simulink model "c00014M_harness"  (R2018a)
settings: Solver=FixedStepAuto  StartTime=0.0  StopTime=300  FixedStep=0.1  RelTol=1e-3
undefined symbols (not defined in the file): A1, hmax, PriorityTank, R1, R2, sigbuilder_block
(part 9 of 24)

== system c00014M_harness/M236/Tank3 ==
  CT3 : Inport
  T3 : Inport  Port=2
  EB3 : Inport  Port=3
  LL1 : Inport  Port=4
  Control : Subsystem
  Logical Operator : Logic  AllPortsSameDT=off  OutDataTypeStr=boolean
  MasterTankControl : Subsystem
  Memory : Memory
  Memory1 : Memory
  TankModel : Subsystem
  LL3 : Outport
  wires:
  TankModel/1(LiquidLevel) -> Memory/1, LL3/1
  Control/1(LiquidIn) -> Logical Operator/1
  Control/2(LiquidOut) -> TankModel/2(LiquidOut)
  Memory/1 -> MasterTankControl/2(LiquidTank3), Control/4(LiquidLevel)
  CT3/1 -> Control/2(StartMaintenance), Control/1(ControlType)
  Memory1/1 -> MasterTankControl/1(LiquidTank1)
  EB3/1 -> Control/3(EmergencyButton)
  MasterTankControl/1(AllowTheTankFilling) -> Logical Operator/2
  Logical Operator/1 -> TankModel/1(LiquidIn)
  LL1/1 -> Memory1/1

== system c00014M_harness/M237/Tank1 ==
  CT1 : Inport
  F1 : Inport  Port=2
  E1 : Inport  Port=3
  T1 : Inport  Port=4
  EB1 : Inport  Port=5
  LL3 : Inport  Port=6
  Control : Subsystem
  Logical Operator : Logic  AllPortsSameDT=off  OutDataTypeStr=boolean
  MasterTankControl : Subsystem
  Memory : Memory
  Memory2 : Memory
  TankModel : Subsystem
  LL1 : Outport
  wires:
  TankModel/1(LiquidLevel) -> Memory/1, LL1/1
  Control/1(LiquidIn) -> Logical Operator/1
  Control/2(LiquidOut) -> TankModel/2(LiquidOut)
  Memory/1 -> Control/5(LiquidLevel), MasterTankControl/1(LiquidTank1)
  CT1/1 -> Control/1(ControlType)
  F1/1 -> Control/2(Fill)
  E1/1 -> Control/3(Empty)
  LL3/1 -> Memory2/1
  Memory2/1 -> MasterTankControl/2(LiquidTank3)
  EB1/1 -> Control/4(EmergencyButton)
  MasterTankControl/1(AllowTheTankFilling) -> Logical Operator/2
  Logical Operator/1 -> TankModel/1(LiquidIn)

== system c00014M_harness/M237/Tank3 ==
  CT3 : Inport
  T3 : Inport  Port=2
  EB3 : Inport  Port=3
  LL1 : Inport  Port=4
  Control : Subsystem
  Logical Operator : Logic  AllPortsSameDT=off  OutDataTypeStr=boolean
  MasterTankControl : Subsystem
  Memory : Memory
  Memory1 : Memory
  TankModel : Subsystem
  LL3 : Outport
  wires:
  TankModel/1(LiquidLevel) -> Memory/1, LL3/1
  Control/1(LiquidIn) -> Logical Operator/1
  Control/2(LiquidOut) -> TankModel/2(LiquidOut)
  Memory/1 -> MasterTankControl/2(LiquidTank3), Control/4(LiquidLevel)
  CT3/1 -> Control/2(StartMaintenance), Control/1(ControlType)
  Memory1/1 -> MasterTankControl/1(LiquidTank1)
  EB3/1 -> Control/3(EmergencyButton)
  MasterTankControl/1(AllowTheTankFilling) -> Logical Operator/2
  Logical Operator/1 -> TankModel/1(LiquidIn)
  LL1/1 -> Memory1/1

== system c00014M_harness/M238/Tank1 ==
  CT1 : Inport
  F1 : Inport  Port=2
  E1 : Inport  Port=3
  T1 : Inport  Port=4
  EB1 : Inport  Port=5
  LL3 : Inport  Port=6
  Control : Subsystem
  Logical Operator : Logic  AllPortsSameDT=off  OutDataTypeStr=boolean
  MasterTankControl : Subsystem
  Memory : Memory
  Memory2 : Memory
  TankModel : Subsystem
  LL1 : Outport
  wires:
  TankModel/1(LiquidLevel) -> Memory/1, LL1/1
  Control/1(LiquidIn) -> Logical Operator/1
  Control/2(LiquidOut) -> TankModel/2(LiquidOut)
  Memory/1 -> Control/5(LiquidLevel), MasterTankControl/1(LiquidTank1)
  CT1/1 -> Control/1(ControlType)
  F1/1 -> Control/2(Fill)
  E1/1 -> Control/3(Empty)
  LL3/1 -> Memory2/1
  Memory2/1 -> MasterTankControl/2(LiquidTank3)
  EB1/1 -> Control/4(EmergencyButton)
  MasterTankControl/1(AllowTheTankFilling) -> Logical Operator/2
  Logical Operator/1 -> TankModel/1(LiquidIn)

== system c00014M_harness/M238/Tank3 ==
  CT3 : Inport
  T3 : Inport  Port=2
  EB3 : Inport  Port=3
  LL1 : Inport  Port=4
  Control : Subsystem
  Logical Operator : Logic  AllPortsSameDT=off  OutDataTypeStr=boolean
  MasterTankControl : Subsystem
  Memory : Memory
  Memory1 : Memory
  TankModel : Subsystem
  LL3 : Outport
  wires:
  TankModel/1(LiquidLevel) -> Memory/1, LL3/1
  Control/1(LiquidIn) -> Logical Operator/1
  Control/2(LiquidOut) -> TankModel/2(LiquidOut)
  Memory/1 -> MasterTankControl/2(LiquidTank3), Control/4(LiquidLevel)
  CT3/1 -> Control/2(StartMaintenance), Control/1(ControlType)
  Memory1/1 -> MasterTankControl/1(LiquidTank1)
  EB3/1 -> Control/3(EmergencyButton)
  MasterTankControl/1(AllowTheTankFilling) -> Logical Operator/2
  Logical Operator/1 -> TankModel/1(LiquidIn)
  LL1/1 -> Memory1/1

== system c00014M_harness/M239/Tank1 ==
  CT1 : Inport
  F1 : Inport  Port=2
  E1 : Inport  Port=3
  T1 : Inport  Port=4
  EB1 : Inport  Port=5
  LL3 : Inport  Port=6
  Control : Subsystem
  Logical Operator : Logic  AllPortsSameDT=off  OutDataTypeStr=boolean
  MasterTankControl : Subsystem
  Memory : Memory
  Memory2 : Memory
  TankModel : Subsystem
  LL1 : Outport
  wires:
  TankModel/1(LiquidLevel) -> Memory/1, LL1/1
  Control/1(LiquidIn) -> Logical Operator/1
  Control/2(LiquidOut) -> TankModel/2(LiquidOut)
  Memory/1 -> Control/5(LiquidLevel), MasterTankControl/1(LiquidTank1)
  CT1/1 -> Control/1(ControlType)
  F1/1 -> Control/2(Fill)
  E1/1 -> Control/3(Empty)
  LL3/1 -> Memory2/1
  Memory2/1 -> MasterTankControl/2(LiquidTank3)
  EB1/1 -> Control/4(EmergencyButton)
  MasterTankControl/1(AllowTheTankFilling) -> Logical Operator/2
  Logical Operator/1 -> TankModel/1(LiquidIn)

== system c00014M_harness/M239/Tank3 ==
  CT3 : Inport
  T3 : Inport  Port=2
  EB3 : Inport  Port=3
  LL1 : Inport  Port=4
  Control : Subsystem
  Logical Operator : Logic  AllPortsSameDT=off  OutDataTypeStr=boolean
  MasterTankControl : Subsystem
  Memory : Memory
  Memory1 : Memory
  TankModel : Subsystem
  LL3 : Outport
  wires:
  TankModel/1(LiquidLevel) -> Memory/1, LL3/1
  Control/1(LiquidIn) -> Logical Operator/1
  Control/2(LiquidOut) -> TankModel/2(LiquidOut)
  Memory/1 -> MasterTankControl/2(LiquidTank3), Control/4(LiquidLevel)
  CT3/1 -> Control/2(StartMaintenance), Control/1(ControlType)
  Memory1/1 -> MasterTankControl/1(LiquidTank1)
  EB3/1 -> Control/3(EmergencyButton)
  MasterTankControl/1(AllowTheTankFilling) -> Logical Operator/2
  Logical Operator/1 -> TankModel/1(LiquidIn)
  LL1/1 -> Memory1/1

== system c00014M_harness/M240/Tank1 ==
  CT1 : Inport
  F1 : Inport  Port=2
  E1 : Inport  Port=3
  T1 : Inport  Port=4
  EB1 : Inport  Port=5
  LL3 : Inport  Port=6
  Control : Subsystem
  Logical Operator : Logic  AllPortsSameDT=off  OutDataTypeStr=boolean
  MasterTankControl : Subsystem
  Memory : Memory
  Memory2 : Memory
  TankModel : Subsystem
  LL1 : Outport
  wires:
  TankModel/1(LiquidLevel) -> Memory/1, LL1/1
  Control/1(LiquidIn) -> Logical Operator/1
  Control/2(LiquidOut) -> TankModel/2(LiquidOut)
  Memory/1 -> Control/5(LiquidLevel), MasterTankControl/1(LiquidTank1)
  CT1/1 -> Control/1(ControlType)
  F1/1 -> Control/2(Fill)
  E1/1 -> Control/3(Empty)
  LL3/1 -> Memory2/1
  Memory2/1 -> MasterTankControl/2(LiquidTank3)
  EB1/1 -> Control/4(EmergencyButton)
  MasterTankControl/1(AllowTheTankFilling) -> Logical Operator/2
  Logical Operator/1 -> TankModel/1(LiquidIn)

== system c00014M_harness/M240/Tank3 ==
  CT3 : Inport
  T3 : Inport  Port=2
  EB3 : Inport  Port=3
  LL1 : Inport  Port=4
  Control : Subsystem
  Logical Operator : Logic  AllPortsSameDT=off  OutDataTypeStr=boolean
  MasterTankControl : Subsystem
  Memory : Memory
  Memory1 : Memory
  TankModel : Subsystem
  LL3 : Outport
  wires:
  TankModel/1(LiquidLevel) -> Memory/1, LL3/1
  Control/1(LiquidIn) -> Logical Operator/1
  Control/2(LiquidOut) -> TankModel/2(LiquidOut)
  Memory/1 -> MasterTankControl/2(LiquidTank3), Control/4(LiquidLevel)
  CT3/1 -> Control/2(StartMaintenance), Control/1(ControlType)
  Memory1/1 -> MasterTankControl/1(LiquidTank1)
  EB3/1 -> Control/3(EmergencyButton)
  MasterTankControl/1(AllowTheTankFilling) -> Logical Operator/2
  Logical Operator/1 -> TankModel/1(LiquidIn)
  LL1/1 -> Memory1/1

== system c00014M_harness/M241/Tank1 ==
  CT1 : Inport
  F1 : Inport  Port=2
  E1 : Inport  Port=3
  T1 : Inport  Port=4
  EB1 : Inport  Port=5
  LL3 : Inport  Port=6
  Control : Subsystem
  Logical Operator : Logic  AllPortsSameDT=off  OutDataTypeStr=boolean
  MasterTankControl : Subsystem
  Memory : Memory
  Memory2 : Memory
  TankModel : Subsystem
  LL1 : Outport
  wires:
  TankModel/1(LiquidLevel) -> Memory/1, LL1/1
  Control/1(LiquidIn) -> Logical Operator/1
  Control/2(LiquidOut) -> TankModel/2(LiquidOut)
  Memory/1 -> Control/5(LiquidLevel), MasterTankControl/1(LiquidTank1)
  CT1/1 -> Control/1(ControlType)
  F1/1 -> Control/2(Fill)
  E1/1 -> Control/3(Empty)
  LL3/1 -> Memory2/1
  Memory2/1 -> MasterTankControl/2(LiquidTank3)
  EB1/1 -> Control/4(EmergencyButton)
  MasterTankControl/1(AllowTheTankFilling) -> Logical Operator/2
  Logical Operator/1 -> TankModel/1(LiquidIn)

== system c00014M_harness/M241/Tank3 ==
  CT3 : Inport
  T3 : Inport  Port=2
  EB3 : Inport  Port=3
  LL1 : Inport  Port=4
  Control : Subsystem
  Logical Operator : Logic  AllPortsSameDT=off  OutDataTypeStr=boolean
  MasterTankControl : Subsystem
  Memory : Memory
  Memory1 : Memory
  TankModel : Subsystem
  LL3 : Outport
  wires:
  TankModel/1(LiquidLevel) -> Memory/1, LL3/1
  Control/1(LiquidIn) -> Logical Operator/1
  Control/2(LiquidOut) -> TankModel/2(LiquidOut)
  Memory/1 -> MasterTankControl/2(LiquidTank3), Control/4(LiquidLevel)
  CT3/1 -> Control/2(StartMaintenance), Control/1(ControlType)
  Memory1/1 -> MasterTankControl/1(LiquidTank1)
  EB3/1 -> Control/3(EmergencyButton)
  MasterTankControl/1(AllowTheTankFilling) -> Logical Operator/2
  Logical Operator/1 -> TankModel/1(LiquidIn)
  LL1/1 -> Memory1/1

== system c00014M_harness/M242/Tank1 ==
  CT1 : Inport
  F1 : Inport  Port=2
  E1 : Inport  Port=3
  T1 : Inport  Port=4
  EB1 : Inport  Port=5
  LL3 : Inport  Port=6
  Control : Subsystem
  Logical Operator : Logic  AllPortsSameDT=off  OutDataTypeStr=boolean
  MasterTankControl : Subsystem
  Memory : Memory
  Memory2 : Memory
  TankModel : Subsystem
  LL1 : Outport
  wires:
  TankModel/1(LiquidLevel) -> Memory/1, LL1/1
  Control/1(LiquidIn) -> Logical Operator/1
  Control/2(LiquidOut) -> TankModel/2(LiquidOut)
  Memory/1 -> Control/5(LiquidLevel), MasterTankControl/1(LiquidTank1)
  CT1/1 -> Control/1(ControlType)
  F1/1 -> Control/2(Fill)
  E1/1 -> Control/3(Empty)
  LL3/1 -> Memory2/1
  Memory2/1 -> MasterTankControl/2(LiquidTank3)
  EB1/1 -> Control/4(EmergencyButton)
  MasterTankControl/1(AllowTheTankFilling) -> Logical Operator/2
  Logical Operator/1 -> TankModel/1(LiquidIn)

== system c00014M_harness/M242/Tank3 ==
  CT3 : Inport
  T3 : Inport  Port=2
  EB3 : Inport  Port=3
  LL1 : Inport  Port=4
  Control : Subsystem
  Logical Operator : Logic  AllPortsSameDT=off  OutDataTypeStr=boolean
  MasterTankControl : Subsystem
  Memory : Memory
  Memory1 : Memory
  TankModel : Subsystem
  LL3 : Outport
  wires:
  TankModel/1(LiquidLevel) -> Memory/1, LL3/1
  Control/1(LiquidIn) -> Logical Operator/1
  Control/2(LiquidOut) -> TankModel/2(LiquidOut)
  Memory/1 -> MasterTankControl/2(LiquidTank3), Control/4(LiquidLevel)
  CT3/1 -> Control/2(StartMaintenance), Control/1(ControlType)
  Memory1/1 -> MasterTankControl/1(LiquidTank1)
  EB3/1 -> Control/3(EmergencyButton)
  MasterTankControl/1(AllowTheTankFilling) -> Logical Operator/2
  Logical Operator/1 -> TankModel/1(LiquidIn)
  LL1/1 -> Memory1/1

== system c00014M_harness/M243/Tank1 ==
  CT1 : Inport
  F1 : Inport  Port=2
  E1 : Inport  Port=3
  T1 : Inport  Port=4
  EB1 : Inport  Port=5
  LL3 : Inport  Port=6
  Control : Subsystem
  Logical Operator : Logic  AllPortsSameDT=off  OutDataTypeStr=boolean
  MasterTankControl : Subsystem
  Memory : Memory
  Memory2 : Memory
  TankModel : Subsystem
  LL1 : Outport
  wires:
  TankModel/1(LiquidLevel) -> Memory/1, LL1/1
  Control/1(LiquidIn) -> Logical Operator/1
  Control/2(LiquidOut) -> TankModel/2(LiquidOut)
  Memory/1 -> Control/5(LiquidLevel), MasterTankControl/1(LiquidTank1)
  CT1/1 -> Control/1(ControlType)
  F1/1 -> Control/2(Fill)
  E1/1 -> Control/3(Empty)
  LL3/1 -> Memory2/1
  Memory2/1 -> MasterTankControl/2(LiquidTank3)
  EB1/1 -> Control/4(EmergencyButton)
  MasterTankControl/1(AllowTheTankFilling) -> Logical Operator/2
  Logical Operator/1 -> TankModel/1(LiquidIn)

== system c00014M_harness/M243/Tank3 ==
  CT3 : Inport
  T3 : Inport  Port=2
  EB3 : Inport  Port=3
  LL1 : Inport  Port=4
  Control : Subsystem
  Logical Operator : Logic  AllPortsSameDT=off  OutDataTypeStr=boolean
  MasterTankControl : Subsystem
  Memory : Memory
  Memory1 : Memory
  TankModel : Subsystem
  LL3 : Outport
  wires:
  TankModel/1(LiquidLevel) -> Memory/1, LL3/1
  Control/1(LiquidIn) -> Logical Operator/1
  Control/2(LiquidOut) -> TankModel/2(LiquidOut)
  Memory/1 -> MasterTankControl/2(LiquidTank3), Control/4(LiquidLevel)
  CT3/1 -> Control/2(StartMaintenance), Control/1(ControlType)
  Memory1/1 -> MasterTankControl/1(LiquidTank1)
  EB3/1 -> Control/3(EmergencyButton)
  MasterTankControl/1(AllowTheTankFilling) -> Logical Operator/2
  Logical Operator/1 -> TankModel/1(LiquidIn)
  LL1/1 -> Memory1/1

== system c00014M_harness/M244/Tank1 ==
  CT1 : Inport
  F1 : Inport  Port=2
  E1 : Inport  Port=3
  T1 : Inport  Port=4
  EB1 : Inport  Port=5
  LL3 : Inport  Port=6
  Control : Subsystem
  Logical Operator : Logic  AllPortsSameDT=off  OutDataTypeStr=boolean
  MasterTankControl : Subsystem
  Memory : Memory
  Memory2 : Memory
  TankModel : Subsystem
  LL1 : Outport
  wires:
  TankModel/1(LiquidLevel) -> Memory/1, LL1/1
  Control/1(LiquidIn) -> Logical Operator/1
  Control/2(LiquidOut) -> TankModel/2(LiquidOut)
  Memory/1 -> Control/5(LiquidLevel), MasterTankControl/1(LiquidTank1)
  CT1/1 -> Control/1(ControlType)
  F1/1 -> Control/2(Fill)
  E1/1 -> Control/3(Empty)
  LL3/1 -> Memory2/1
  Memory2/1 -> MasterTankControl/2(LiquidTank3)
  EB1/1 -> Control/4(EmergencyButton)
  MasterTankControl/1(AllowTheTankFilling) -> Logical Operator/2
  Logical Operator/1 -> TankModel/1(LiquidIn)

== system c00014M_harness/M244/Tank3 ==
  CT3 : Inport
  T3 : Inport  Port=2
  EB3 : Inport  Port=3
  LL1 : Inport  Port=4
  Control : Subsystem
  Logical Operator : Logic  AllPortsSameDT=off  OutDataTypeStr=boolean
  MasterTankControl : Subsystem
  Memory : Memory
  Memory1 : Memory
  TankModel : Subsystem
  LL3 : Outport
  wires:
  TankModel/1(LiquidLevel) -> Memory/1, LL3/1
  Control/1(LiquidIn) -> Logical Operator/1
  Control/2(LiquidOut) -> TankModel/2(LiquidOut)
  Memory/1 -> MasterTankControl/2(LiquidTank3), Control/4(LiquidLevel)
  CT3/1 -> Control/2(StartMaintenance), Control/1(ControlType)
  Memory1/1 -> MasterTankControl/1(LiquidTank1)
  EB3/1 -> Control/3(EmergencyButton)
  MasterTankControl/1(AllowTheTankFilling) -> Logical Operator/2
  Logical Operator/1 -> TankModel/1(LiquidIn)
  LL1/1 -> Memory1/1

== system c00014M_harness/M245/Tank1 ==
  CT1 : Inport
  F1 : Inport  Port=2
  E1 : Inport  Port=3
  T1 : Inport  Port=4
  EB1 : Inport  Port=5
  LL3 : Inport  Port=6
  Control : Subsystem
  Logical Operator : Logic  AllPortsSameDT=off  OutDataTypeStr=boolean
  MasterTankControl : Subsystem
  Memory : Memory
  Memory2 : Memory
  TankModel : Subsystem
  LL1 : Outport
  wires:
  TankModel/1(LiquidLevel) -> Memory/1, LL1/1
  Control/1(LiquidIn) -> Logical Operator/1
  Control/2(LiquidOut) -> TankModel/2(LiquidOut)
  Memory/1 -> Control/5(LiquidLevel), MasterTankControl/1(LiquidTank1)
  CT1/1 -> Control/1(ControlType)
  F1/1 -> Control/2(Fill)
  E1/1 -> Control/3(Empty)
  LL3/1 -> Memory2/1
  Memory2/1 -> MasterTankControl/2(LiquidTank3)
  EB1/1 -> Control/4(EmergencyButton)
  MasterTankControl/1(AllowTheTankFilling) -> Logical Operator/2
  Logical Operator/1 -> TankModel/1(LiquidIn)

== system c00014M_harness/M245/Tank3 ==
  CT3 : Inport
  T3 : Inport  Port=2
  EB3 : Inport  Port=3
  LL1 : Inport  Port=4
  Control : Subsystem
  Logical Operator : Logic  AllPortsSameDT=off  OutDataTypeStr=boolean
  MasterTankControl : Subsystem
  Memory : Memory
  Memory1 : Memory
  TankModel : Subsystem
  LL3 : Outport
  wires:
  TankModel/1(LiquidLevel) -> Memory/1, LL3/1
  Control/1(LiquidIn) -> Logical Operator/1
  Control/2(LiquidOut) -> TankModel/2(LiquidOut)
  Memory/1 -> MasterTankControl/2(LiquidTank3), Control/4(LiquidLevel)
  CT3/1 -> Control/2(StartMaintenance), Control/1(ControlType)
  Memory1/1 -> MasterTankControl/1(LiquidTank1)
  EB3/1 -> Control/3(EmergencyButton)
  MasterTankControl/1(AllowTheTankFilling) -> Logical Operator/2
  Logical Operator/1 -> TankModel/1(LiquidIn)
  LL1/1 -> Memory1/1

== system c00014M_harness/M246/Tank1 ==
  CT1 : Inport
  F1 : Inport  Port=2
  E1 : Inport  Port=3
  T1 : Inport  Port=4
  EB1 : Inport  Port=5
  LL3 : Inport  Port=6
  Control : Subsystem
  Logical Operator : Logic  AllPortsSameDT=off  OutDataTypeStr=boolean
  MasterTankControl : Subsystem
  Memory : Memory
  Memory2 : Memory
  TankModel : Subsystem
  LL1 : Outport
  wires:
  TankModel/1(LiquidLevel) -> Memory/1, LL1/1
  Control/1(LiquidIn) -> Logical Operator/1
  Control/2(LiquidOut) -> TankModel/2(LiquidOut)
  Memory/1 -> Control/5(LiquidLevel), MasterTankControl/1(LiquidTank1)
  CT1/1 -> Control/1(ControlType)
  F1/1 -> Control/2(Fill)
  E1/1 -> Control/3(Empty)
  LL3/1 -> Memory2/1
  Memory2/1 -> MasterTankControl/2(LiquidTank3)
  EB1/1 -> Control/4(EmergencyButton)
  MasterTankControl/1(AllowTheTankFilling) -> Logical Operator/2
  Logical Operator/1 -> TankModel/1(LiquidIn)

== system c00014M_harness/M246/Tank3 ==
  CT3 : Inport
  T3 : Inport  Port=2
  EB3 : Inport  Port=3
  LL1 : Inport  Port=4
  Control : Subsystem
  Logical Operator : Logic  AllPortsSameDT=off  OutDataTypeStr=boolean
  MasterTankControl : Subsystem
  Memory : Memory
  Memory1 : Memory
  TankModel : Subsystem
  LL3 : Outport
  wires:
  TankModel/1(LiquidLevel) -> Memory/1, LL3/1
  Control/1(LiquidIn) -> Logical Operator/1
  Control/2(LiquidOut) -> TankModel/2(LiquidOut)
  Memory/1 -> MasterTankControl/2(LiquidTank3), Control/4(LiquidLevel)
  CT3/1 -> Control/2(StartMaintenance), Control/1(ControlType)
  Memory1/1 -> MasterTankControl/1(LiquidTank1)
  EB3/1 -> Control/3(EmergencyButton)
  MasterTankControl/1(AllowTheTankFilling) -> Logical Operator/2
  Logical Operator/1 -> TankModel/1(LiquidIn)
  LL1/1 -> Memory1/1

== system c00014M_harness/CPSUT/Tank1/Control ==
  note: 1: Maintenance
      | 2: Reference
      | 3: Manual
  ControlType : Inport
  Fill : Inport  Port=2
  Empty : Inport  Port=3
  EmergencyButton : Inport  Port=4
  LiquidLevel : Inport  Port=5
  Constant : Constant  Value=0
  ManualControlLiquidInOut : Subsystem
  Switch : Switch  Criteria=u2 > Threshold
  Switch1 : Switch  Criteria=u2 > Threshold
  LiquidIn : Outport
  LiquidOut : Outport  Port=2
  wires:
  LiquidLevel/1 -> ManualControlLiquidInOut/3(LiquidLevel)
  Empty/1 -> ManualControlLiquidInOut/2(Empty)
  Fill/1 -> ManualControlLiquidInOut/1(Fill)
  Switch/1 -> LiquidIn/1
  Switch1/1 -> LiquidOut/1
  Constant/1 -> Switch1/1, Switch/1
  EmergencyButton/1 -> Switch/2, Switch1/2
  ManualControlLiquidInOut/1(LiquidIn) -> Switch/3
  ManualControlLiquidInOut/2(LiquidOut) -> Switch1/3

== system c00014M_harness/CPSUT/Tank1/MasterTankControl ==
  note: Priority tank must always have more liquid than others
  LiquidTank1 : Inport
  LiquidTank3 : Inport  Port=2
  Constant : Constant  Value=PriorityTank
  Constant1 : Constant  Value=false
  Logical Operator : Logic  Operator=NOT  AllPortsSameDT=off  OutDataTypeStr=boolean
  Multiport Switch : MultiPortSwitch
  Relational Operator1 : RelationalOperator  OutDataTypeStr=boolean  RndMeth=Simplest
  AllowTheTankFilling : Outport
  wires:
  LiquidTank3/1 -> Relational Operator1/2
  LiquidTank1/1 -> Relational Operator1/1
  Constant/1 -> Multiport Switch/1
  Relational Operator1/1 -> Multiport Switch/4
  Constant1/1 -> Multiport Switch/2, Multiport Switch/3
  Multiport Switch/1 -> Logical Operator/1
  Logical Operator/1 -> AllowTheTankFilling/1

== system c00014M_harness/CPSUT/Tank1/TankModel ==
  LiquidIn : Inport
  LiquidOut : Inport  Port=2
  Add1 : Sum  Inputs=+-
  Constant1 : Constant  Value=0
  Constant2 : Constant  Value=0
  Constant3 : Constant
  Gain : Gain  Gain=1/R1
  Gain1 : Gain  Gain=1/A1
  Gain2 : Gain  Gain=1/R2
  Integrator : Integrator
  Saturation : Saturate  UpperLimit=hmax  LowerLimit=0
  Switch : Switch  Criteria=u2 ~= 0
  Switch1 : Switch  Criteria=u2 ~= 0
  LiquidLevel : Outport
  wires:
  Saturation/1 -> LiquidLevel/1, Gain2/1
  LiquidOut/1 -> Switch/2
  Add1/1 -> Gain1/1
  Gain2/1 -> Switch/1
  LiquidIn/1 -> Switch1/2
  Switch/1 -> Add1/2
  Switch1/1 -> Gain/1
  Constant2/1 -> Switch/3
  Constant3/1 -> Switch1/1
  Integrator/1 -> Saturation/1
  Gain1/1 -> Integrator/1
  Gain/1 -> Add1/1
  Constant1/1 -> Switch1/3

== system c00014M_harness/CPSUT/Tank3/Control ==
  note: 1: Maintenance
      | 2: Reference
      | 3: Manual
  ControlType : Inport
  StartMaintenance : Inport  Port=2
  EmergencyButton : Inport  Port=3
  LiquidLevel : Inport  Port=4
  Constant : Constant  Value=0
  Maintenance : Subsystem
  Switch : Switch  Criteria=u2 > Threshold
  Switch1 : Switch  Criteria=u2 > Threshold
  LiquidIn : Outport
  LiquidOut : Outport  Port=2
  wires:
  ControlType/1 -> Maintenance/1(Type)
  LiquidLevel/1 -> Maintenance/3(LiquidLevel)
  StartMaintenance/1 -> Maintenance/2(StartMaintenance)
  Switch/1 -> LiquidIn/1
  Switch1/1 -> LiquidOut/1
  Constant/1 -> Switch1/1, Switch/1
  EmergencyButton/1 -> Switch/2, Switch1/2
  Maintenance/1(LiquidIn) -> Switch/3
  Maintenance/2(LiquidOut) -> Switch1/3

== system c00014M_harness/CPSUT/Tank3/MasterTankControl ==
  note: Priority tank must always have more liquid than others
  LiquidTank1 : Inport
  LiquidTank3 : Inport  Port=2
  Constant : Constant  Value=PriorityTank
  Constant1 : Constant  Value=false
  Logical Operator : Logic  Operator=NOT  AllPortsSameDT=off  OutDataTypeStr=boolean
  Multiport Switch : MultiPortSwitch
  Relational Operator : RelationalOperator  OutDataTypeStr=boolean  RndMeth=Simplest
  AllowTheTankFilling : Outport
  wires:
  Constant/1 -> Multiport Switch/1
  Relational Operator/1 -> Multiport Switch/2
  Constant1/1 -> Multiport Switch/4, Multiport Switch/3
  Multiport Switch/1 -> Logical Operator/1
  Logical Operator/1 -> AllowTheTankFilling/1
  LiquidTank1/1 -> Relational Operator/2
  LiquidTank3/1 -> Relational Operator/1

== system c00014M_harness/CPSUT/Tank3/TankModel ==
  LiquidIn : Inport
  LiquidOut : Inport  Port=2
  Add1 : Sum  Inputs=+-
  Constant1 : Constant  Value=0
  Constant2 : Constant  Value=0
  Constant3 : Constant
  Gain : Gain  Gain=1/R1
  Gain1 : Gain  Gain=1/A1
  Gain2 : Gain  Gain=1/R2
  Integrator : Integrator
  Saturation : Saturate  UpperLimit=hmax  LowerLimit=0
  Switch : Switch  Criteria=u2 ~= 0
  Switch1 : Switch  Criteria=u2 ~= 0
  LiquidLevel : Outport
  wires:
  Saturation/1 -> LiquidLevel/1, Gain2/1
  LiquidOut/1 -> Switch/2
  Add1/1 -> Gain1/1
  Gain2/1 -> Switch/1
  LiquidIn/1 -> Switch1/2
  Switch/1 -> Add1/2
  Switch1/1 -> Gain/1
  Constant2/1 -> Switch/3
  Constant3/1 -> Switch1/1
  Integrator/1 -> Saturation/1
  Gain1/1 -> Integrator/1
  Gain/1 -> Add1/1
  Constant1/1 -> Switch1/3

== system c00014M_harness/M001/Tank1/Control ==
  note: 1: Maintenance
      | 2: Reference
      | 3: Manual
  ControlType : Inport
  Fill : Inport  Port=2
  Empty : Inport  Port=3
  EmergencyButton : Inport  Port=4
  LiquidLevel : Inport  Port=5
  Constant : Constant
  ManualControlLiquidInOut : Subsystem
  Switch : Switch  Criteria=u2 > Threshold
  Switch1 : Switch  Criteria=u2 > Threshold
  LiquidIn : Outport
  LiquidOut : Outport  Port=2
  wires:
  Constant/1 -> Switch/1, Switch1/1
  Switch1/1 -> LiquidOut/1
  Switch/1 -> LiquidIn/1
  Fill/1 -> ManualControlLiquidInOut/1(Fill)
  Empty/1 -> ManualControlLiquidInOut/2(Empty)
  LiquidLevel/1 -> ManualControlLiquidInOut/3(LiquidLevel)
  EmergencyButton/1 -> Switch/2, Switch1/2
  ManualControlLiquidInOut/1(LiquidIn) -> Switch/3
  ManualControlLiquidInOut/2(LiquidOut) -> Switch1/3

== system c00014M_harness/M001/Tank1/MasterTankControl ==
  note: Priority tank must always have more liquid than others
  LiquidTank1 : Inport
  LiquidTank3 : Inport  Port=2
  Constant : Constant  Value=PriorityTank
  Constant1 : Constant  Value=false
  Logical Operator : Logic  Operator=NOT  AllPortsSameDT=off  OutDataTypeStr=boolean
  Multiport Switch : MultiPortSwitch
  Relational Operator1 : RelationalOperator  OutDataTypeStr=boolean  RndMeth=Simplest
  AllowTheTankFilling : Outport
  wires:
  Logical Operator/1 -> AllowTheTankFilling/1
  Multiport Switch/1 -> Logical Operator/1
  Constant1/1 -> Multiport Switch/2, Multiport Switch/3
  Relational Operator1/1 -> Multiport Switch/4
  Constant/1 -> Multiport Switch/1
  LiquidTank1/1 -> Relational Operator1/1
  LiquidTank3/1 -> Relational Operator1/2

== system c00014M_harness/M001/Tank1/TankModel ==
  LiquidIn : Inport
  LiquidOut : Inport  Port=2
  Add1 : Sum  Inputs=+-
  Constant1 : Constant  Value=0
  Constant2 : Constant  Value=0
  Constant3 : Constant
  Gain : Gain  Gain=1/R1
  Gain1 : Gain  Gain=1/A1
  Gain2 : Gain  Gain=1/R2
  Integrator : Integrator
  Saturation : Saturate  UpperLimit=hmax  LowerLimit=0
  Switch : Switch  Criteria=u2 ~= 0
  Switch1 : Switch  Criteria=u2 ~= 0
  LiquidLevel : Outport
  wires:
  Constant1/1 -> Switch1/3
  Gain/1 -> Add1/1
  Gain1/1 -> Integrator/1
  Integrator/1 -> Saturation/1
  Constant3/1 -> Switch1/1
  Constant2/1 -> Switch/3
  Switch1/1 -> Gain/1
  Switch/1 -> Add1/2
  LiquidIn/1 -> Switch1/2
  Gain2/1 -> Switch/1
  Add1/1 -> Gain1/1
  LiquidOut/1 -> Switch/2
  Saturation/1 -> Gain2/1, LiquidLevel/1

== system c00014M_harness/M001/Tank3/Control ==
  note: 1: Maintenance
      | 2: Reference
      | 3: Manual
  ControlType : Inport
  StartMaintenance : Inport  Port=2
  EmergencyButton : Inport  Port=3
  LiquidLevel : Inport  Port=4
  Constant : Constant  Value=0
  Maintenance : Subsystem
  Switch : Switch  Criteria=u2 > Threshold
  Switch1 : Switch  Criteria=u2 > Threshold
  LiquidIn : Outport
  LiquidOut : Outport  Port=2
  wires:
  Constant/1 -> Switch/1, Switch1/1
  Switch1/1 -> LiquidOut/1
  Switch/1 -> LiquidIn/1
  StartMaintenance/1 -> Maintenance/2(StartMaintenance)
  LiquidLevel/1 -> Maintenance/3(LiquidLevel)
  ControlType/1 -> Maintenance/1(Type)
  EmergencyButton/1 -> Switch/2, Switch1/2
  Maintenance/1(LiquidIn) -> Switch/3
  Maintenance/2(LiquidOut) -> Switch1/3

== system c00014M_harness/M001/Tank3/MasterTankControl ==
  note: Priority tank must always have more liquid than others
  LiquidTank1 : Inport
  LiquidTank3 : Inport  Port=2
  Constant : Constant  Value=PriorityTank
  Constant1 : Constant  Value=false
  Logical Operator : Logic  Operator=NOT  AllPortsSameDT=off  OutDataTypeStr=boolean
  Multiport Switch : MultiPortSwitch
  Relational Operator : RelationalOperator  OutDataTypeStr=boolean  RndMeth=Simplest
  AllowTheTankFilling : Outport
  wires:
  LiquidTank3/1 -> Relational Operator/1
  LiquidTank1/1 -> Relational Operator/2
  Logical Operator/1 -> AllowTheTankFilling/1
  Multiport Switch/1 -> Logical Operator/1
  Constant1/1 -> Multiport Switch/4, Multiport Switch/3
  Relational Operator/1 -> Multiport Switch/2
  Constant/1 -> Multiport Switch/1

== system c00014M_harness/M001/Tank3/TankModel ==
  LiquidIn : Inport
  LiquidOut : Inport  Port=2
  Add1 : Sum  Inputs=+-
  Constant1 : Constant  Value=0
  Constant2 : Constant  Value=0
  Constant3 : Constant
  Gain : Gain  Gain=1/R1
  Gain1 : Gain  Gain=1/A1
  Gain2 : Gain  Gain=1/R2
  Integrator : Integrator
  Saturation : Saturate  UpperLimit=hmax  LowerLimit=0
  Switch : Switch  Criteria=u2 ~= 0
  Switch1 : Switch  Criteria=u2 ~= 0
  LiquidLevel : Outport
  wires:
  Constant1/1 -> Switch1/3
  Gain/1 -> Add1/1
  Gain1/1 -> Integrator/1
  Integrator/1 -> Saturation/1
  Constant3/1 -> Switch1/1
  Constant2/1 -> Switch/3
  Switch1/1 -> Gain/1
  Switch/1 -> Add1/2
  LiquidIn/1 -> Switch1/2
  Gain2/1 -> Switch/1
  Add1/1 -> Gain1/1
  LiquidOut/1 -> Switch/2
  Saturation/1 -> Gain2/1, LiquidLevel/1

== system c00014M_harness/M036/Tank1/Control ==
  note: 1: Maintenance
      | 2: Reference
      | 3: Manual
  ControlType : Inport
  Fill : Inport  Port=2
  Empty : Inport  Port=3
  EmergencyButton : Inport  Port=4
  LiquidLevel : Inport  Port=5
  Constant : Constant  Value=0
  ManualControlLiquidInOut : Subsystem
  Switch : Switch  Criteria=u2 > Threshold
  Switch1 : Switch  Criteria=u2 > Threshold
  LiquidIn : Outport
  LiquidOut : Outport  Port=2
  wires:
  LiquidLevel/1 -> ManualControlLiquidInOut/3(LiquidLevel)
  Empty/1 -> ManualControlLiquidInOut/2(Empty)
  Fill/1 -> ManualControlLiquidInOut/1(Fill)
  Switch/1 -> LiquidIn/1
  Switch1/1 -> LiquidOut/1
  Constant/1 -> Switch1/1, Switch/1
  EmergencyButton/1 -> Switch/2, Switch1/2
  ManualControlLiquidInOut/1(LiquidIn) -> Switch/3
  ManualControlLiquidInOut/2(LiquidOut) -> Switch1/3

== system c00014M_harness/M036/Tank1/MasterTankControl ==
  note: Priority tank must always have more liquid than others
  LiquidTank1 : Inport
  LiquidTank3 : Inport  Port=2
  Constant : Constant  Value=PriorityTank
  Constant1 : Constant  Value=false
  Logical Operator : Logic  Operator=NOT  AllPortsSameDT=off  OutDataTypeStr=boolean
  Multiport Switch : MultiPortSwitch
  Relational Operator1 : RelationalOperator  OutDataTypeStr=boolean  RndMeth=Simplest
  AllowTheTankFilling : Outport
  wires:
  LiquidTank3/1 -> Relational Operator1/2
  LiquidTank1/1 -> Relational Operator1/1
  Constant/1 -> Multiport Switch/1
  Relational Operator1/1 -> Multiport Switch/4
  Constant1/1 -> Multiport Switch/2, Multiport Switch/3
  Multiport Switch/1 -> Logical Operator/1
  Logical Operator/1 -> AllowTheTankFilling/1

== system c00014M_harness/M036/Tank1/TankModel ==
  LiquidIn : Inport
  LiquidOut : Inport  Port=2
  Add1 : Sum  Inputs=+-
  Constant1 : Constant  Value=0
  Constant2 : Constant  Value=0
  Constant3 : Constant
  Gain : Gain  Gain=1/R1
  Gain1 : Gain  Gain=1/A1
  Gain2 : Gain  Gain=1/R2
  Integrator : Integrator
  Saturation : Saturate  UpperLimit=hmax  LowerLimit=0
  Switch : Switch  Criteria=u2 ~= 0
  Switch1 : Switch  Criteria=u2 ~= 0
  LiquidLevel : Outport
  wires:
  Saturation/1 -> LiquidLevel/1, Gain2/1
  LiquidOut/1 -> Switch/2
  Add1/1 -> Gain1/1
  Gain2/1 -> Switch/1
  LiquidIn/1 -> Switch1/2
  Switch/1 -> Add1/2
  Switch1/1 -> Gain/1
  Constant2/1 -> Switch/3
  Constant3/1 -> Switch1/1
  Integrator/1 -> Saturation/1
  Gain1/1 -> Integrator/1
  Gain/1 -> Add1/1
  Constant1/1 -> Switch1/3

== system c00014M_harness/M036/Tank3/Control ==
  note: 1: Maintenance
      | 2: Reference
      | 3: Manual
  ControlType : Inport
  StartMaintenance : Inport  Port=2
  EmergencyButton : Inport  Port=3
  LiquidLevel : Inport  Port=4
  Constant : Constant  Value=0
  Maintenance : Subsystem
  Switch : Switch  Criteria=u2 > Threshold
  Switch1 : Switch  Criteria=u2 > Threshold
  LiquidIn : Outport
  LiquidOut : Outport  Port=2
  wires:
  ControlType/1 -> Maintenance/1(Type)
  LiquidLevel/1 -> Maintenance/3(LiquidLevel)
  StartMaintenance/1 -> Maintenance/2(StartMaintenance)
  Switch/1 -> LiquidIn/1
  Switch1/1 -> LiquidOut/1
  Constant/1 -> Switch1/1, Switch/1
  EmergencyButton/1 -> Switch/2, Switch1/2
  Maintenance/1(LiquidIn) -> Switch/3
  Maintenance/2(LiquidOut) -> Switch1/3

== system c00014M_harness/M036/Tank3/MasterTankControl ==
  note: Priority tank must always have more liquid than others
  LiquidTank1 : Inport
  LiquidTank3 : Inport  Port=2
  Constant : Constant  Value=PriorityTank
  Constant1 : Constant  Value=false
  Logical Operator : Logic  Operator=NOT  AllPortsSameDT=off  OutDataTypeStr=boolean
  Multiport Switch : MultiPortSwitch
  Relational Operator : RelationalOperator  OutDataTypeStr=boolean  RndMeth=Simplest
  AllowTheTankFilling : Outport
  wires:
  Constant/1 -> Multiport Switch/1
  Relational Operator/1 -> Multiport Switch/2
  Constant1/1 -> Multiport Switch/4, Multiport Switch/3
  Multiport Switch/1 -> Logical Operator/1
  Logical Operator/1 -> AllowTheTankFilling/1
  LiquidTank1/1 -> Relational Operator/2
  LiquidTank3/1 -> Relational Operator/1

== system c00014M_harness/M036/Tank3/TankModel ==
  LiquidIn : Inport
  LiquidOut : Inport  Port=2
  Add1 : Sum  Inputs=+-
  Constant1 : Constant  Value=0
  Constant2 : Constant  Value=0
  Constant3 : Constant
  Gain : Gain  Gain=1/R1
  Gain1 : Gain  Gain=1/A1
  Gain2 : Gain  Gain=1/R2
  Integrator : Integrator
  Saturation : Saturate  UpperLimit=hmax  LowerLimit=0
  Switch : Switch  Criteria=u2 ~= 0
  Switch1 : Switch  Criteria=u2 ~= 0
  LiquidLevel : Outport
  wires:
  Saturation/1 -> LiquidLevel/1, Gain2/1
  LiquidOut/1 -> Switch/2
  Add1/1 -> Gain1/1
  Gain2/1 -> Switch/1
  LiquidIn/1 -> Switch1/2
  Switch/1 -> Add1/2
  Switch1/1 -> Gain/1
  Constant2/1 -> Switch/3
  Constant3/1 -> Switch1/1
  Integrator/1 -> Saturation/1
  Gain1/1 -> Integrator/1
  Gain/1 -> Add1/1
  Constant1/1 -> Switch1/3

== system c00014M_harness/M037/Tank1/Control ==
  note: 1: Maintenance
      | 2: Reference
      | 3: Manual
  ControlType : Inport
  Fill : Inport  Port=2
  Empty : Inport  Port=3
  EmergencyButton : Inport  Port=4
  LiquidLevel : Inport  Port=5
  Constant : Constant  Value=0
  ManualControlLiquidInOut : Subsystem
  Switch : Switch  Criteria=u2 > Threshold
  Switch1 : Switch  Criteria=u2 > Threshold
  LiquidIn : Outport
  LiquidOut : Outport  Port=2
  wires:
  LiquidLevel/1 -> ManualControlLiquidInOut/3(LiquidLevel)
  Empty/1 -> ManualControlLiquidInOut/2(Empty)
  Fill/1 -> ManualControlLiquidInOut/1(Fill)
  Switch/1 -> LiquidIn/1
  Switch1/1 -> LiquidOut/1
  Constant/1 -> Switch1/1, Switch/1
  EmergencyButton/1 -> Switch/2, Switch1/2
  ManualControlLiquidInOut/1(LiquidIn) -> Switch/3
  ManualControlLiquidInOut/2(LiquidOut) -> Switch1/3

== system c00014M_harness/M037/Tank1/MasterTankControl ==
  note: Priority tank must always have more liquid than others
  LiquidTank1 : Inport
  LiquidTank3 : Inport  Port=2
  Constant : Constant  Value=PriorityTank
  Constant1 : Constant  Value=false
  Logical Operator : Logic  Operator=NOT  AllPortsSameDT=off  OutDataTypeStr=boolean
  Multiport Switch : MultiPortSwitch
  Relational Operator1 : RelationalOperator  OutDataTypeStr=boolean  RndMeth=Simplest
  AllowTheTankFilling : Outport
  wires:
  LiquidTank3/1 -> Relational Operator1/2
  LiquidTank1/1 -> Relational Operator1/1
  Constant/1 -> Multiport Switch/1
  Relational Operator1/1 -> Multiport Switch/4
  Constant1/1 -> Multiport Switch/2, Multiport Switch/3
  Multiport Switch/1 -> Logical Operator/1
  Logical Operator/1 -> AllowTheTankFilling/1

== system c00014M_harness/M037/Tank1/TankModel ==
  LiquidIn : Inport
  LiquidOut : Inport  Port=2
  Add1 : Sum  Inputs=+-
  Constant1 : Constant  Value=0
  Constant2 : Constant  Value=0
  Constant3 : Constant
  Gain : Gain  Gain=1/R1
  Gain1 : Gain  Gain=1/A1
  Gain2 : Gain  Gain=1/R2
  Integrator : Integrator
  Saturation : Saturate  UpperLimit=hmax  LowerLimit=0
  Switch : Switch  Criteria=u2 ~= 0
  Switch1 : Switch  Criteria=u2 ~= 0
  LiquidLevel : Outport
  wires:
  Saturation/1 -> LiquidLevel/1, Gain2/1
  LiquidOut/1 -> Switch/2
  Add1/1 -> Gain1/1
  Gain2/1 -> Switch/1
  LiquidIn/1 -> Switch1/2
  Switch/1 -> Add1/2
  Switch1/1 -> Gain/1
  Constant2/1 -> Switch/3
  Constant3/1 -> Switch1/1
  Integrator/1 -> Saturation/1
  Gain1/1 -> Integrator/1
  Gain/1 -> Add1/1
  Constant1/1 -> Switch1/3

== system c00014M_harness/M037/Tank3/Control ==
  note: 1: Maintenance
      | 2: Reference
      | 3: Manual
  ControlType : Inport
  StartMaintenance : Inport  Port=2
  EmergencyButton : Inport  Port=3
  LiquidLevel : Inport  Port=4
  Constant : Constant  Value=0
  Maintenance : Subsystem
  Switch : Switch  Criteria=u2 > Threshold
  Switch1 : Switch  Criteria=u2 > Threshold
  LiquidIn : Outport
  LiquidOut : Outport  Port=2
  wires:
  ControlType/1 -> Maintenance/1(Type)
  LiquidLevel/1 -> Maintenance/3(LiquidLevel)
  StartMaintenance/1 -> Maintenance/2(StartMaintenance)
  Switch/1 -> LiquidIn/1
  Switch1/1 -> LiquidOut/1
  Constant/1 -> Switch1/1, Switch/1
  EmergencyButton/1 -> Switch/2, Switch1/2
  Maintenance/1(LiquidIn) -> Switch/3
  Maintenance/2(LiquidOut) -> Switch1/3

== system c00014M_harness/M037/Tank3/MasterTankControl ==
  note: Priority tank must always have more liquid than others
  LiquidTank1 : Inport
  LiquidTank3 : Inport  Port=2
  Constant : Constant  Value=PriorityTank
  Constant1 : Constant  Value=false
  Logical Operator : Logic  Operator=NOT  AllPortsSameDT=off  OutDataTypeStr=boolean
  Multiport Switch : MultiPortSwitch
  Relational Operator : RelationalOperator  OutDataTypeStr=boolean  RndMeth=Simplest
  AllowTheTankFilling : Outport
  wires:
  Constant/1 -> Multiport Switch/1
  Relational Operator/1 -> Multiport Switch/2
  Constant1/1 -> Multiport Switch/4, Multiport Switch/3
  Multiport Switch/1 -> Logical Operator/1
  Logical Operator/1 -> AllowTheTankFilling/1
  LiquidTank1/1 -> Relational Operator/2
  LiquidTank3/1 -> Relational Operator/1

== system c00014M_harness/M037/Tank3/TankModel ==
  LiquidIn : Inport
  LiquidOut : Inport  Port=2
  Add1 : Sum  Inputs=+-
  Constant1 : Constant  Value=0
  Constant2 : Constant  Value=0
  Constant3 : Constant
  Gain : Gain  Gain=1/R1
  Gain1 : Gain  Gain=1/A1
  Gain2 : Gain  Gain=1/R2
  Integrator : Integrator
  Saturation : Saturate  UpperLimit=hmax  LowerLimit=0
  Switch : Switch  Criteria=u2 ~= 0
  Switch1 : Switch  Criteria=u2 ~= 0
  LiquidLevel : Outport
  wires:
  Saturation/1 -> LiquidLevel/1, Gain2/1
  LiquidOut/1 -> Switch/2
  Add1/1 -> Gain1/1
  Gain2/1 -> Switch/1
  LiquidIn/1 -> Switch1/2
  Switch/1 -> Add1/2
  Switch1/1 -> Gain/1
  Constant2/1 -> Switch/3
  Constant3/1 -> Switch1/1
  Integrator/1 -> Saturation/1
  Gain1/1 -> Integrator/1
  Gain/1 -> Add1/1
  Constant1/1 -> Switch1/3

== system c00014M_harness/M038/Tank1/Control ==
  note: 1: Maintenance
      | 2: Reference
      | 3: Manual
  ControlType : Inport
  Fill : Inport  Port=2
  Empty : Inport  Port=3
  EmergencyButton : Inport  Port=4
  LiquidLevel : Inport  Port=5
  Constant : Constant  Value=0
  ManualControlLiquidInOut : Subsystem
  Switch : Switch  Criteria=u2 > Threshold
  Switch1 : Switch  Criteria=u2 > Threshold
  LiquidIn : Outport
  LiquidOut : Outport  Port=2
  wires:
  LiquidLevel/1 -> ManualControlLiquidInOut/3(LiquidLevel)
  Empty/1 -> ManualControlLiquidInOut/2(Empty)
  Fill/1 -> ManualControlLiquidInOut/1(Fill)
  Switch/1 -> LiquidIn/1
  Switch1/1 -> LiquidOut/1
  Constant/1 -> Switch1/1, Switch/1
  EmergencyButton/1 -> Switch/2, Switch1/2
  ManualControlLiquidInOut/1(LiquidIn) -> Switch/3
  ManualControlLiquidInOut/2(LiquidOut) -> Switch1/3

== system c00014M_harness/M038/Tank1/MasterTankControl ==
  note: Priority tank must always have more liquid than others
  LiquidTank1 : Inport
  LiquidTank3 : Inport  Port=2
  Constant : Constant  Value=PriorityTank
  Constant1 : Constant  Value=false
  Logical Operator : Logic  Operator=NOT  AllPortsSameDT=off  OutDataTypeStr=boolean
  Multiport Switch : MultiPortSwitch
  Relational Operator1 : RelationalOperator  OutDataTypeStr=boolean  RndMeth=Simplest
  AllowTheTankFilling : Outport
  wires:
  LiquidTank3/1 -> Relational Operator1/2
  LiquidTank1/1 -> Relational Operator1/1
  Constant/1 -> Multiport Switch/1
  Relational Operator1/1 -> Multiport Switch/4
  Constant1/1 -> Multiport Switch/2, Multiport Switch/3
  Multiport Switch/1 -> Logical Operator/1
  Logical Operator/1 -> AllowTheTankFilling/1

== system c00014M_harness/M038/Tank1/TankModel ==
  LiquidIn : Inport
  LiquidOut : Inport  Port=2
  Add1 : Sum  Inputs=+-
  Constant1 : Constant  Value=0
  Constant2 : Constant  Value=0
  Constant3 : Constant
  Gain : Gain  Gain=1/R1
  Gain1 : Gain  Gain=1/A1
  Gain2 : Gain  Gain=1/R2
  Integrator : Integrator
  Saturation : Saturate  UpperLimit=hmax  LowerLimit=0
  Switch : Switch  Criteria=u2 ~= 0
  Switch1 : Switch  Criteria=u2 ~= 0
  LiquidLevel : Outport
  wires:
  Saturation/1 -> LiquidLevel/1, Gain2/1
  LiquidOut/1 -> Switch/2
  Add1/1 -> Gain1/1
  Gain2/1 -> Switch/1
  LiquidIn/1 -> Switch1/2
  Switch/1 -> Add1/2
  Switch1/1 -> Gain/1
  Constant2/1 -> Switch/3
  Constant3/1 -> Switch1/1
  Integrator/1 -> Saturation/1
  Gain1/1 -> Integrator/1
  Gain/1 -> Add1/1
  Constant1/1 -> Switch1/3

== system c00014M_harness/M038/Tank3/Control ==
  note: 1: Maintenance
      | 2: Reference
      | 3: Manual
  ControlType : Inport
  StartMaintenance : Inport  Port=2
  EmergencyButton : Inport  Port=3
  LiquidLevel : Inport  Port=4
  Constant : Constant  Value=0
  Maintenance : Subsystem
  Switch : Switch  Criteria=u2 > Threshold
  Switch1 : Switch  Criteria=u2 > Threshold
  LiquidIn : Outport
  LiquidOut : Outport  Port=2
  wires:
  ControlType/1 -> Maintenance/1(Type)
  LiquidLevel/1 -> Maintenance/3(LiquidLevel)
  StartMaintenance/1 -> Maintenance/2(StartMaintenance)
  Switch/1 -> LiquidIn/1
  Switch1/1 -> LiquidOut/1
  Constant/1 -> Switch1/1, Switch/1
  EmergencyButton/1 -> Switch/2, Switch1/2
  Maintenance/1(LiquidIn) -> Switch/3
  Maintenance/2(LiquidOut) -> Switch1/3

== system c00014M_harness/M038/Tank3/MasterTankControl ==
  note: Priority tank must always have more liquid than others
  LiquidTank1 : Inport
  LiquidTank3 : Inport  Port=2
  Constant : Constant  Value=PriorityTank
  Constant1 : Constant  Value=false
  Logical Operator : Logic  Operator=NOT  AllPortsSameDT=off  OutDataTypeStr=boolean
  Multiport Switch : MultiPortSwitch
  Relational Operator : RelationalOperator  OutDataTypeStr=boolean  RndMeth=Simplest
  AllowTheTankFilling : Outport
  wires:
  Constant/1 -> Multiport Switch/1
  Relational Operator/1 -> Multiport Switch/2
  Constant1/1 -> Multiport Switch/4, Multiport Switch/3
  Multiport Switch/1 -> Logical Operator/1
  Logical Operator/1 -> AllowTheTankFilling/1
  LiquidTank1/1 -> Relational Operator/2
  LiquidTank3/1 -> Relational Operator/1

== system c00014M_harness/M038/Tank3/TankModel ==
  LiquidIn : Inport
  LiquidOut : Inport  Port=2
  Add1 : Sum  Inputs=+-
  Constant1 : Constant  Value=0
  Constant2 : Constant  Value=0
  Constant3 : Constant
  Gain : Gain  Gain=1/R1
  Gain1 : Gain  Gain=1/A1
  Gain2 : Gain  Gain=1/R2
  Integrator : Integrator
  Saturation : Saturate  UpperLimit=hmax  LowerLimit=0
  Switch : Switch  Criteria=u2 ~= 0
  Switch1 : Switch  Criteria=u2 ~= 0
  LiquidLevel : Outport
  wires:
  Saturation/1 -> LiquidLevel/1, Gain2/1
  LiquidOut/1 -> Switch/2
  Add1/1 -> Gain1/1
  Gain2/1 -> Switch/1
  LiquidIn/1 -> Switch1/2
  Switch/1 -> Add1/2
  Switch1/1 -> Gain/1
  Constant2/1 -> Switch/3
  Constant3/1 -> Switch1/1
  Integrator/1 -> Saturation/1
  Gain1/1 -> Integrator/1
  Gain/1 -> Add1/1
  Constant1/1 -> Switch1/3

== system c00014M_harness/M039/Tank1/Control ==
  note: 1: Maintenance
      | 2: Reference
      | 3: Manual
  ControlType : Inport
  Fill : Inport  Port=2
  Empty : Inport  Port=3
  EmergencyButton : Inport  Port=4
  LiquidLevel : Inport  Port=5
  Constant : Constant  Value=0
  ManualControlLiquidInOut : Subsystem
  Switch : Switch  Criteria=u2 > Threshold
  Switch1 : Switch  Criteria=u2 > Threshold
  LiquidIn : Outport
  LiquidOut : Outport  Port=2
  wires:
  LiquidLevel/1 -> ManualControlLiquidInOut/3(LiquidLevel)
  Empty/1 -> ManualControlLiquidInOut/2(Empty)
  Fill/1 -> ManualControlLiquidInOut/1(Fill)
  Switch/1 -> LiquidIn/1
  Switch1/1 -> LiquidOut/1
  Constant/1 -> Switch1/1, Switch/1
  EmergencyButton/1 -> Switch/2, Switch1/2
  ManualControlLiquidInOut/1(LiquidIn) -> Switch/3
  ManualControlLiquidInOut/2(LiquidOut) -> Switch1/3

== system c00014M_harness/M039/Tank1/MasterTankControl ==
  note: Priority tank must always have more liquid than others
  LiquidTank1 : Inport
  LiquidTank3 : Inport  Port=2
  Constant : Constant  Value=PriorityTank
  Constant1 : Constant  Value=false
  Logical Operator : Logic  Operator=NOT  AllPortsSameDT=off  OutDataTypeStr=boolean
  Multiport Switch : MultiPortSwitch
  Relational Operator1 : RelationalOperator  OutDataTypeStr=boolean  RndMeth=Simplest
  AllowTheTankFilling : Outport
  wires:
  LiquidTank3/1 -> Relational Operator1/2
  LiquidTank1/1 -> Relational Operator1/1
  Constant/1 -> Multiport Switch/1
  Relational Operator1/1 -> Multiport Switch/4
  Constant1/1 -> Multiport Switch/2, Multiport Switch/3
  Multiport Switch/1 -> Logical Operator/1
  Logical Operator/1 -> AllowTheTankFilling/1

== system c00014M_harness/M039/Tank1/TankModel ==
  LiquidIn : Inport
  LiquidOut : Inport  Port=2
  Add1 : Sum  Inputs=+-
  Constant1 : Constant  Value=0
  Constant2 : Constant  Value=0
  Constant3 : Constant
  Gain : Gain  Gain=1/R1
  Gain1 : Gain  Gain=1/A1
  Gain2 : Gain  Gain=1/R2
  Integrator : Integrator
  Saturation : Saturate  UpperLimit=hmax  LowerLimit=0
  Switch : Switch  Criteria=u2 ~= 0
  Switch1 : Switch  Criteria=u2 ~= 0
  LiquidLevel : Outport
  wires:
  Saturation/1 -> LiquidLevel/1, Gain2/1
  LiquidOut/1 -> Switch/2
  Add1/1 -> Gain1/1
  Gain2/1 -> Switch/1
  LiquidIn/1 -> Switch1/2
  Switch/1 -> Add1/2
  Switch1/1 -> Gain/1
  Constant2/1 -> Switch/3
  Constant3/1 -> Switch1/1
  Integrator/1 -> Saturation/1
  Gain1/1 -> Integrator/1
  Gain/1 -> Add1/1
  Constant1/1 -> Switch1/3

== system c00014M_harness/M039/Tank3/Control ==
  note: 1: Maintenance
      | 2: Reference
      | 3: Manual
  ControlType : Inport
  StartMaintenance : Inport  Port=2
  EmergencyButton : Inport  Port=3
  LiquidLevel : Inport  Port=4
  Constant : Constant  Value=0
  Maintenance : Subsystem
  Switch : Switch  Criteria=u2 > Threshold
  Switch1 : Switch  Criteria=u2 > Threshold
  LiquidIn : Outport
  LiquidOut : Outport  Port=2
  wires:
  ControlType/1 -> Maintenance/1(Type)
  LiquidLevel/1 -> Maintenance/3(LiquidLevel)
  StartMaintenance/1 -> Maintenance/2(StartMaintenance)
  Switch/1 -> LiquidIn/1
  Switch1/1 -> LiquidOut/1
  Constant/1 -> Switch1/1, Switch/1
  EmergencyButton/1 -> Switch/2, Switch1/2
  Maintenance/1(LiquidIn) -> Switch/3
  Maintenance/2(LiquidOut) -> Switch1/3

== system c00014M_harness/M039/Tank3/MasterTankControl ==
  note: Priority tank must always have more liquid than others
  LiquidTank1 : Inport
  LiquidTank3 : Inport  Port=2
  Constant : Constant  Value=PriorityTank
  Constant1 : Constant  Value=false
  Logical Operator : Logic  Operator=NOT  AllPortsSameDT=off  OutDataTypeStr=boolean
  Multiport Switch : MultiPortSwitch
  Relational Operator : RelationalOperator  OutDataTypeStr=boolean  RndMeth=Simplest
  AllowTheTankFilling : Outport
  wires:
  Constant/1 -> Multiport Switch/1
  Relational Operator/1 -> Multiport Switch/2
  Constant1/1 -> Multiport Switch/4, Multiport Switch/3
  Multiport Switch/1 -> Logical Operator/1
  Logical Operator/1 -> AllowTheTankFilling/1
  LiquidTank1/1 -> Relational Operator/2
  LiquidTank3/1 -> Relational Operator/1

== system c00014M_harness/M039/Tank3/TankModel ==
  LiquidIn : Inport
  LiquidOut : Inport  Port=2
  Add1 : Sum  Inputs=+-
  Constant1 : Constant  Value=0
  Constant2 : Constant  Value=0
  Constant3 : Constant
  Gain : Gain  Gain=1/R1
  Gain1 : Gain  Gain=1/A1
  Gain2 : Gain  Gain=1/R2
  Integrator : Integrator
  Saturation : Saturate  UpperLimit=hmax  LowerLimit=0
  Switch : Switch  Criteria=u2 ~= 0
  Switch1 : Switch  Criteria=u2 ~= 0
  LiquidLevel : Outport
  wires:
  Saturation/1 -> LiquidLevel/1, Gain2/1
  LiquidOut/1 -> Switch/2
  Add1/1 -> Gain1/1
  Gain2/1 -> Switch/1
  LiquidIn/1 -> Switch1/2
  Switch/1 -> Add1/2
  Switch1/1 -> Gain/1
  Constant2/1 -> Switch/3
  Constant3/1 -> Switch1/1
  Integrator/1 -> Saturation/1
  Gain1/1 -> Integrator/1
  Gain/1 -> Add1/1
  Constant1/1 -> Switch1/3

== system c00014M_harness/M040/Tank1/Control ==
  note: 1: Maintenance
      | 2: Reference
      | 3: Manual
  ControlType : Inport
  Fill : Inport  Port=2
  Empty : Inport  Port=3
  EmergencyButton : Inport  Port=4
  LiquidLevel : Inport  Port=5
  Constant : Constant  Value=0
  ManualControlLiquidInOut : Subsystem
  Switch : Switch  Criteria=u2 > Threshold
  Switch1 : Switch  Criteria=u2 > Threshold
  LiquidIn : Outport
  LiquidOut : Outport  Port=2
  wires:
  LiquidLevel/1 -> ManualControlLiquidInOut/3(LiquidLevel)
  Empty/1 -> ManualControlLiquidInOut/2(Empty)
  Fill/1 -> ManualControlLiquidInOut/1(Fill)
  Switch/1 -> LiquidIn/1
  Switch1/1 -> LiquidOut/1
  Constant/1 -> Switch1/1, Switch/1
  EmergencyButton/1 -> Switch/2, Switch1/2
  ManualControlLiquidInOut/1(LiquidIn) -> Switch/3
  ManualControlLiquidInOut/2(LiquidOut) -> Switch1/3

== system c00014M_harness/M040/Tank1/MasterTankControl ==
  note: Priority tank must always have more liquid than others
  LiquidTank1 : Inport
  LiquidTank3 : Inport  Port=2
  Constant : Constant  Value=PriorityTank
  Constant1 : Constant  Value=false
  Logical Operator : Logic  Operator=NOT  AllPortsSameDT=off  OutDataTypeStr=boolean
  Multiport Switch : MultiPortSwitch
  Relational Operator1 : RelationalOperator  OutDataTypeStr=boolean  RndMeth=Simplest
  AllowTheTankFilling : Outport
  wires:
  LiquidTank3/1 -> Relational Operator1/2
  LiquidTank1/1 -> Relational Operator1/1
  Constant/1 -> Multiport Switch/1
  Relational Operator1/1 -> Multiport Switch/4
  Constant1/1 -> Multiport Switch/2, Multiport Switch/3
  Multiport Switch/1 -> Logical Operator/1
  Logical Operator/1 -> AllowTheTankFilling/1

== system c00014M_harness/M040/Tank1/TankModel ==
  LiquidIn : Inport
  LiquidOut : Inport  Port=2
  Add1 : Sum  Inputs=+-
  Constant1 : Constant  Value=0
  Constant2 : Constant  Value=0
  Constant3 : Constant
  Gain : Gain  Gain=1/R1
  Gain1 : Gain  Gain=1/A1
  Gain2 : Gain  Gain=1/R2
  Integrator : Integrator
  Saturation : Saturate  UpperLimit=hmax  LowerLimit=0
  Switch : Switch  Criteria=u2 ~= 0
  Switch1 : Switch  Criteria=u2 ~= 0
  LiquidLevel : Outport
  wires:
  Saturation/1 -> LiquidLevel/1, Gain2/1
  LiquidOut/1 -> Switch/2
  Add1/1 -> Gain1/1
  Gain2/1 -> Switch/1
  LiquidIn/1 -> Switch1/2
  Switch/1 -> Add1/2
  Switch1/1 -> Gain/1
  Constant2/1 -> Switch/3
  Constant3/1 -> Switch1/1
  Integrator/1 -> Saturation/1
  Gain1/1 -> Integrator/1
  Gain/1 -> Add1/1
  Constant1/1 -> Switch1/3
